simulink model "DPT"  (R2023a)
settings: Solver=VariableStepAuto  StartTime=0.0  StopTime=1  RelTol=1e-3
values from neighbouring files (symbols this model uses):
  J = 0.08    [main.m]
  km = 0.032    [main.m]
  kv = 0.288    [main.m]
  L = 0.4    [main.m]
  R = 0.8    [main.m]
settings Model: Creator=ycheb  LastModifiedBy=ycheb

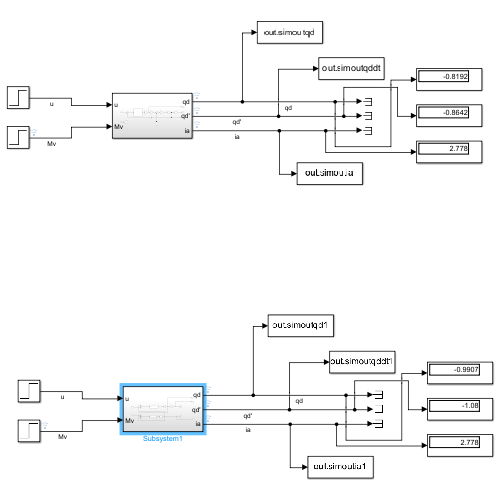
[thumbnail: Simulink's stored preview of the top-level diagram]
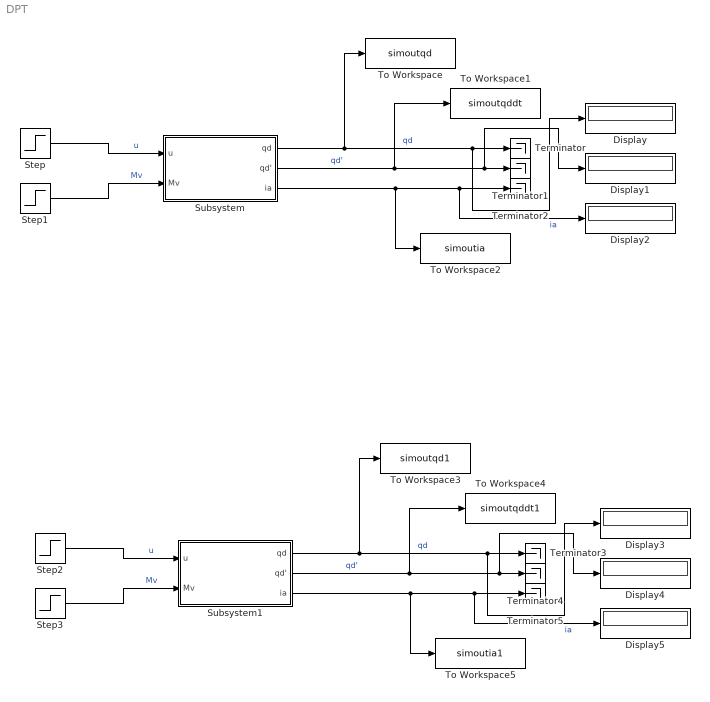
== system DPT ==
  Display{,1..5} (6 alike) : Display
  Step{,1..3} (4 alike) : Step  Time=0  SampleTime=0
  Subsystem : Subsystem
  Subsystem1 : Subsystem
  Terminator{,1..5} (6 alike) : Terminator
  To Workspace : ToWorkspace  VariableName=simoutqd  SaveFormat=Timeseries  SampleTime=-1
  To Workspace1 : ToWorkspace  VariableName=simoutqddt  SaveFormat=Timeseries  SampleTime=-1
  To Workspace2 : ToWorkspace  VariableName=simoutia  SaveFormat=Timeseries  SampleTime=-1
  To Workspace3 : ToWorkspace  VariableName=simoutqd1  SaveFormat=Timeseries  SampleTime=-1
  To Workspace4 : ToWorkspace  VariableName=simoutqddt1  SaveFormat=Timeseries  SampleTime=-1
  To Workspace5 : ToWorkspace  VariableName=simoutia1  SaveFormat=Timeseries  SampleTime=-1
  wires:
  Step/1 -> Subsystem/1(u)  "u"
  Step1/1 -> Subsystem/2(Mv)  "Mv"
  Subsystem/3(ia) -> To Workspace2/1, Display2/1, Terminator2/1  "ia"
  Subsystem/2(qd') -> To Workspace1/1, Display1/1, Terminator1/1  "qd'"
  Subsystem/1(qd) -> To Workspace/1, Display/1, Terminator/1  "qd"
  Subsystem1/3(ia) -> To Workspace5/1, Display5/1, Terminator5/1  "ia"
  Step3/1 -> Subsystem1/2(Mv)  "Mv"
  Subsystem1/2(qd') -> To Workspace4/1, Display4/1, Terminator4/1  "qd'"
  Subsystem1/1(qd) -> To Workspace3/1, Display3/1, Terminator3/1  "qd"
  Step2/1 -> Subsystem1/1(u)  "u"

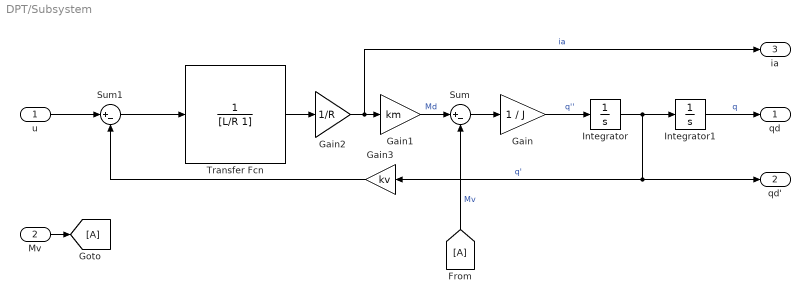
== system DPT/Subsystem ==
  u : Inport
  Mv : Inport  Port=2
  From : From
  Gain : Gain  Gain=1 / J
  Gain1 : Gain  Gain=km
  Gain2 : Gain  Gain=1/R
  Gain3 : Gain  Gain=kv
  Goto : Goto
  Integrator : Integrator
  Integrator1 : Integrator
  Sum : Sum  Inputs=|+-
  Sum1 : Sum  Inputs=|+-
  Transfer Fcn : TransferFcn  Denominator=[L/R 1]
  qd : Outport
  qd' : Outport  Port=2
  ia : Outport  Port=3
  wires:
  Integrator/1 -> qd'/1, Gain3/1, Integrator1/1  "q'"
  Gain/1 -> Integrator/1  "q''"
  Integrator1/1 -> qd/1  "q"
  Sum/1 -> Gain/1
  From/1 -> Sum/2  "Mv"
  Gain1/1 -> Sum/1  "Md"
  u/1 -> Sum1/1
  Gain2/1 -> ia/1, Gain1/1  "ia"
  Transfer Fcn/1 -> Gain2/1
  Gain3/1 -> Sum1/2
  Sum1/1 -> Transfer Fcn/1
  Mv/1 -> Goto/1

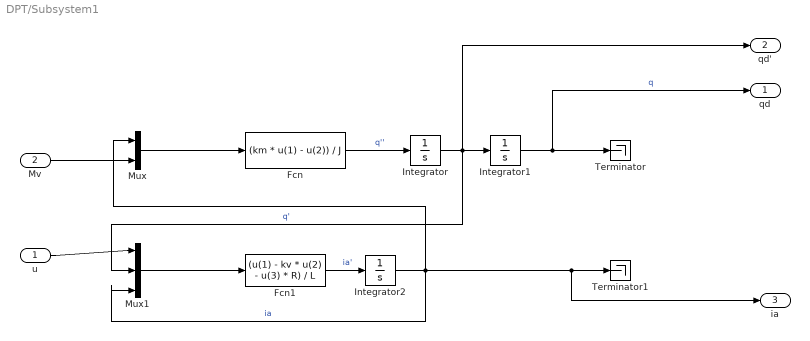
== system DPT/Subsystem1 ==
  u : Inport
  Mv : Inport  Port=2
  Fcn : Fcn  Expr=(km * u(1) - u(2)) / J
  Fcn1 : Fcn  Expr=(u(1) - kv * u(2) - u(3) * R) / L
  Integrator : Integrator
  Integrator1 : Integrator
  Integrator2 : Integrator
  Mux : Mux  Inputs=2
  Mux1 : Mux  Inputs=3
  Terminator : Terminator
  Terminator1 : Terminator
  qd : Outport
  qd' : Outport  Port=2
  ia : Outport  Port=3
  wires:
  Mux/1 -> Fcn/1
  Mv/1 -> Mux/2
  Fcn/1 -> Integrator/1  "q''"
  Integrator2/1 -> Mux1/3, Mux/1, ia/1, Terminator1/1  "ia"
  Integrator/1 -> qd'/1, Mux1/2, Integrator1/1  "q'"
  Integrator1/1 -> qd/1, Terminator/1  "q"
  u/1 -> Mux1/1
  Mux1/1 -> Fcn1/1
  Fcn1/1 -> Integrator2/1  "ia'"
